simulink model "ksp_zad13"  (Simulink 2.20)
settings: Solver=ode45  StartTime=0.0  StopTime=5  RelTol=1e-3  AbsTol=1e-6
settings Model: ConsistencyChecking=off  RTWPlaceOutputsASAP=off

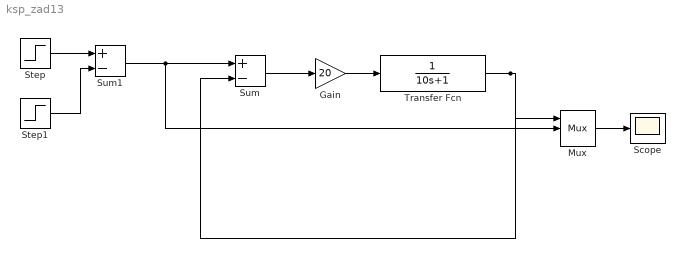
== system ksp_zad13 ==
  Gain : Gain  Gain=20
  Mux : Mux  Inputs=3
  Scope : Scope
      settings: TickLabels=on  TimeRange=5  YMin=-0.05  YMax=1.05  SaveToWorkspace=off  SaveName=ScopeData
  Step : Step  Time=0  Before=0  After=1
  Step1 : Step  Time=1  Before=0  After=1
  Sum : Sum  Inputs=+-
  Sum1 : Sum  Inputs=+-
  Transfer Fcn : TransferFcn  Numerator=[1]  Denominator=[10 1]
  wires:
  Mux/1 -> Scope/1
  Step/1 -> Sum1/1
  Step1/1 -> Sum1/2
  Sum1/1 -> Sum/1, Mux/2
  Gain/1 -> Transfer Fcn/1
  Sum/1 -> Gain/1
  Transfer Fcn/1 -> Sum/2, Mux/1
